simulink model "zad"  (R2016a)
settings: Solver=VariableStepAuto  StartTime=0.0  StopTime=10.0  MaxStep=2^-7  RelTol=1e-3
settings Model: Creator=sk42595  LastModifiedBy=sk42595

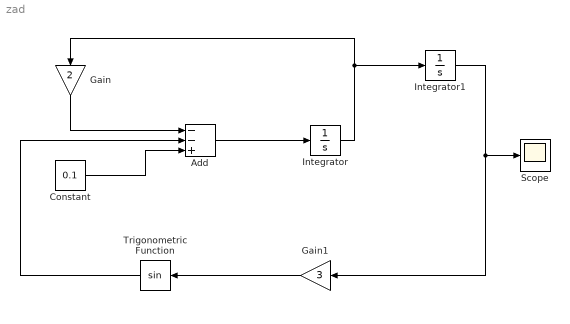
== system zad ==
  Add : Sum  Inputs=--+
  Constant : Constant  Value=0.1
  Gain : Gain  Gain=2
  Gain1 : Gain  Gain=3
  Integrator : Integrator  InitialCondition=2
  Integrator1 : Integrator
  Scope : Scope
  Trigonometric Function : Trigonometry
  wires:
  Integrator/1 -> Integrator1/1, Gain/1
  Add/1 -> Integrator/1
  Constant/1 -> Add/3
  Gain/1 -> Add/1
  Integrator1/1 -> Gain1/1, Scope/1
  Gain1/1 -> Trigonometric Function/1
  Trigonometric Function/1 -> Add/2
